simulink model "csthl20_control"  (R2022a)
settings: Solver=ode45  StartTime=0.0  StopTime=80  RelTol=1e-3  EnableMultiTasking=on
PreLoadFcn:
  | % Bus objects
  | load csthl20_BusData
  | 
  | % Controller configuration
  | CTYPE=1;
model workspace (MAT data in the model file):
  A_matrix = [-0.028840208852 -0.0156596305643 -0.0560912779756 -0.0863202941854 0.0209519994416 0.0112571762889 0 0 0 0 0 0 ... (11560 elements, 17x17x8x5)]
  Act2Aero = [0.5 0.5 0 0 0 0 -0.5 0.5 0 0 0 0 ... (42 elements, 6x7)]
  Aero2Act = [1 -1 0 0 0 0 0 1 1 0 0 0 ... (42 elements, 7x6)]
  Aimpoint = 0
  B_matrix = [0 0 0 0 0 0 4 0 0 0 0 0 ... (2040 elements, 17x3x8x5)]
  CX0 = [-0.038092388 -0.040074629 -0.041654124 -0.043173149 -0.044873204 -0.046895013 -0.049278524 -0.051962909 -0.054786564 -0.057487109 -0.059701388 -0.057487109 ... (861 elements, 21x41)]
  CXda = [0.0003742 1.961503e-05 -0.00027008192 -0.00050147477 -0.00068084192 -0.00081415625 -0.00090708512 -0.00096499037 -0.00099292832 -0.00099564977 -0.0009776 -0.00094291877 ... (41 elements, 41x1)]
  CXddf = [0.00027645 0.00032803699 0.00037408304 0.00041515629 0.00045179224 0.00048449375 0.00051373104 0.00053994169 0.00056353064 0.00058487019 0.0006043 0.00062212709 ... (41 elements, 41x1)]
  CXde = [0.00044324 0.000381836538 0.000331656768 0.000291344258 0.000259608768 0.00023522625 0.000217038848 0.000203954898 0.000194948928 0.000189061658 0.0001854 0.000183137058 ... (41 elements, 41x1)]
  CXdfn = [0.00044751 0.0004427177 0.0004388568 0.0004359273 0.0004339292 0.0004328625 0.0004327272 0.0004335233 0.0004352508 0.0004379097 0.0004415 0.0004460217 ... (41 elements, 41x1)]
  CXdfp = [-0.0001151958 -0.000116790098 -0.000118381312 -0.000119969442 -0.000121554488 -0.00012313645 -0.000124715328 -0.000126291122 -0.000127863832 -0.000129433458 -0.000131 -0.000132563458 ... (41 elements, 41x1)]
  CXdr = [0.00020501 3.1047221e-05 -0.000113321344 -0.000231591139 -0.000327061744 -0.000402836875 -0.000461824384 -0.000506736259 -0.000540088624 -0.000564201739 -0.0005812 -0.000593011939 ... (41 elements, 41x1)]
  CYbeta = -0.01242
  CYda = [0.003136571 0.0031983806691 0.0032503278976 0.0032928109331 0.0033262201776 0.0033509381875 0.0033673396736 0.0033757915011 0.0033766526896 0.0033702744131 0.003357 0.0033371649331 ... (41 elements, 41x1)]
  CYddf = [0.000435181 0.0003943016261 0.0003529648896 0.0003113622901 0.0002696754896 0.0002280763125 0.0001867267456 0.0001457789381 0.0001053752016 6.56480101e-05 2.672e-05 -1.12960299e-05 ... (41 elements, 41x1)]
  CYdr = [0.00252708114 0.00237481862595 0.00224430427494 0.00213447047171 0.00204424955574 0.00197257382125 0.00191837551718 0.00188058684723 0.00185813996982 0.00184996699811 0.001855 0.00187217099811 ... (41 elements, 41x1)]
  CZ0 = [0.4485479 0.452540024 0.457747164 0.464172584 0.471737564 0.4802814 0.489561404 0.499252904 0.508949244 0.518161784 0.5263199 0.518161784 ... (861 elements, 21x41)]
  CZda = [0.00078435 0.000747062965 0.00070172464 0.000650226765 0.00059433784 0.000535703125 0.00047584464 0.000416161165 0.00035792824 0.000302298165 0.0002503 0.000202839565 ... (41 elements, 41x1)]
  CZde = [-0.004135092 -0.004296890179 -0.00444395712 -0.004576811367 -0.004695912448 -0.004801660875 -0.004894398144 -0.004974406735 -0.005041910112 -0.005097072723 -0.00514 -0.005170738359 ... (41 elements, 41x1)]
  CZdfn = [-0.00344578 -0.003560437128 -0.003648409408 -0.003712592248 -0.003755747808 -0.003780505 -0.003789359488 -0.003784673688 -0.003768676768 -0.003743464648 -0.003711 -0.003673112248 ... (41 elements, 41x1)]
  CZdfp = [-0.003786031 -0.00378532664 -0.00378462256 -0.00378391876 -0.00378321524 -0.003782512 -0.00378180904 -0.00378110636 -0.00378040396 -0.00377970184 -0.003779 -0.00377829844 ... (41 elements, 41x1)]
  CZdr = [-0.0005037 -0.00036015136 -0.00026716816 -0.00021701736 -0.00020244976 -0.0002167 -0.00025348656 -0.00030701176 -0.00037196176 -0.00044350656 -0.0005173 -0.00058947976 ... (41 elements, 41x1)]
  C_matrix = [0 0 0 0 0 0 0 0 0 -58.994812472 0 0 ... (2040 elements, 3x17x8x5)]
  Clbeta = -0.00787
  Clda = [0.001932032 0.0020326391442 0.0021237120512 0.0022054993322 0.0022782453312 0.002342190125 0.0023975695232 0.0024446150682 0.0024835540352 0.0025146094322 0.002538 0.0025539402122 ... (41 elements, 41x1)]
  Clddf = [0.0007872 0.000807745996 0.000820040096 0.000825228156 0.000824391616 0.0008185475 0.000808648416 0.000795582556 0.000780173696 0.000763181196 0.0007453 0.000727160636 ... (41 elements, 41x1)]
  Cldr = [0.00131521 0.001082613421 0.000885702656 0.000721130461 0.000585704656 0.000476388125 0.000390298816 0.000324709741 0.000277048976 0.000244899661 0.000226 0.000218243261 ... (41 elements, 41x1)]
  Clp = [-0.498 -0.6 -0.398 -0.579 -0.425 -0.499 -0.649 -0.619 -0.81 -0.872 -2.41]
  Clr = [0.496 0.598 0.84 0.806 0.686 0.572 0.603 0.899 0.957 1.357 4.49]
  Cm0 = [0.0380742 0.038701881 0.039695376 0.040900701 0.042196056 0.043491825 0.044730576 0.045887061 0.046968216 0.048013161 0.0490932 0.048013161 ... (861 elements, 21x41)]
  Cmda = [-0.00172492 -0.001358222162 -0.001043014432 -0.000774578842 -0.000548407232 -0.00036020125 -0.000205872352 -8.1541802e-05 1.6459328e-05 9.1590158e-05 0.0001471 0.000186028358 ... (41 elements, 41x1)]
  Cmde = [-0.00155002 -0.001596102826 -0.001641310016 -0.001685002906 -0.001726581856 -0.00176548625 -0.001801194496 -0.001833224026 -0.001861131296 -0.001884511786 -0.001903 -0.001916269466 ... (41 elements, 41x1)]
  Cmdfn = [-0.00114421 -0.001160648097 -0.001169150592 -0.001170952777 -0.001167224592 -0.001159070625 -0.001147530112 -0.001133576937 -0.001118119632 -0.001102001377 -0.001086 -0.001070827977 ... (41 elements, 41x1)]
  Cmdfp = [-0.000989578757 -0.00098958144857 -0.00098958401408 -0.00098958645353 -0.00098958876692 -0.00098959095425 -0.00098959301552 -0.00098959495073 -0.00098959675988 -0.00098959844297 -0.0009896 -0.00098960143097 ... (41 elements, 41x1)]
  Cmdr = [0.000290283 0.0002382539513 0.0001902563968 0.0001463019633 0.0001063833968 7.04745625e-05 3.85304448e-05 1.04871473e-05 -1.37381072e-05 -3.42469767e-05 -5.116e-05 -6.46165967e-05 ... (41 elements, 41x1)]
  Cmq = [-0.203 -0.158 -0.116 -0.176 -0.176 -0.175 -0.174 -0.252 -0.299 -0.571 -0.8]
  Cn0 = [0 0 0 0 0 0 0 0 0 0.0046 0.0056 0.01 ... (36 elements, 9x4)]
  Cnda = [-0.00092498 -0.001272671988 -0.001576223168 -0.001838775908 -0.002063359968 -0.0022528925 -0.002410178048 -0.002537908548 -0.002638663328 -0.002714909108 -0.002769 -0.002803177508 ... (41 elements, 41x1)]
  Cnddf = [-0.000146484 -0.0001398019207 -0.0001321750752 -0.0001237254087 -0.0001145714752 -0.0001048284375 -9.46080672e-05 -8.40187447e-05 -7.31654592e-05 -6.21498087e-05 -5.107e-05 -4.00208487e-05 ... (41 elements, 41x1)]
  Cndr = [-0.0021525 -0.00197387964 -0.00182075584 -0.00169102464 -0.00158266224 -0.001493725 -0.00142234944 -0.00136675224 -0.00132523024 -0.00129616044 -0.001278 -0.00126928624 ... (41 elements, 41x1)]
  Cnp = [0.381 0.353 0.219 0.244 0.179 0.167 0.201 0.222 0.307 0.379 0.85]
  Cnr = [-0.794 -0.837 -0.921 -0.922 -0.867 -0.922 -0.946 -1.007 -1.09 -1.286 -2.041]
  Euler_0 = [0; -0.199448681609; 0.174532925199]
  F_matrix = [5.97622599319 0.726116013193 -2.64604157338 40.7494939461 -11.661494324 -21.0342779763 -20.6745716213 19.9416021106 13.12545371 -926.002157715 187.969629212 231.434488107 ... (2040 elements, 3x17x8x5)]
  H_matrix = [-0.0157218860845 -0.283968320777 0.321370128412 0.271058535159 0.0185568065093 -0.00784369239396 -0.320886300542 1.82463546416 -0.0471251877299 0.142152392032 -0.0609086167769 0.505612659091 ... (2040 elements, 17x3x8x5)]
  Inertia = [12429.9503379  0  0; 0  72478.3946274  0; 0  0  72478.3946274]
  Ixx = 12429.9503379
  Iyy = 72478.3946274
  Izz = 72478.3946274
  Kalpha = [0.0423424456751 0.0568591289308 0.102067434202 0.0770570952411 0.0850957010804 0.0662889030912 0.0515945392978 0.0567349800611 0.0609882520612 0.0639334226074 0.102956303686 0.0735712249771 ... (40 elements, 8x5)]
  Kalpha_1 = [0.0675525766417; 0.0670941520285; 0.105277724217; 0.0705938909254; 0.0692391670282; 0.0682506457138; 0.0672739862702; 0.0668102273189]
  Kbeta = [-0.0421966217034 -0.0316770241418 -0.0293493744968 -0.0256527675357 -0.0307095576987 -0.0325234533837 -0.0335699630482 -0.0320760010348 -0.034523712176 -0.0332114192463 -0.0353203051713 -0.0341700804254 ... (40 elements, 8x5)]
  Kbeta_1 = [-0.0493656538568; -0.0419788515038; -0.0374619432887; -0.0381850673629; -0.0395050518916; -0.0416555062349; -0.0442775778109; -0.0483706672557]
  Kg2lb = 2.20462
  Kg2slug = 0.0685218
  Ki33 = [0.05 0 0 0 0.05 0 0 0 -0.05 0.05 0 0 ... (360 elements, 3x3x8x5)]
  Kp = [58.994812472 52.4118047689 51.4724972494 52.6814724048 55.5352541837 58.9018334743 63.6260316602 72.5872875233 59.9420490209 52.6642968779 51.592012551 53.0773749012 ... (40 elements, 8x5)]
  Kp_1 = [60.2253428509; 52.7939261692; 51.6224369342; 53.1835874806; 55.9559014793; 59.5393657693; 64.8225348547; 75.6927037235]
  Kphi = [0.0897851430865 0.0905292361524 0.0908849236023 0.0911263381707 0.0895187966623 0.0900454862025 0.0906744952369 0.0929073813074 0.0903130708487 0.090501875878 0.0906948768638 0.0909697583395 ... (40 elements, 8x5)]
  Kphi_1 = [0.0899736559878; 0.0903144259517; 0.0907381573489; 0.0909707194509; 0.0897040590713; 0.0897346237436; 0.0909239286068; 0.092390635977]
  Kq = [-180.388522844 -183.274455652 -174.601566615 -173.806564517 -181.332040221 -198.869769941 -229.860472425 -279.151066798 -195.144174655 -181.815188811 -174.318203455 -173.650391198 ... (40 elements, 8x5)]
  Kq_1 = [-190.665384898; -180.322553126; -174.03272401; -173.493656781; -180.877109643; -197.917252796; -228.270830002; -278.51108854]
  Kr = [-713.893478208 -1002.12341186 -1153.7416491 -1153.7295441 -1077.83714501 -1007.5234901 -1017.22971433 -1059.1938939 -717.84572737 -1002.7104968 -1155.32550182 -1152.14420545 ... (40 elements, 8x5)]
  Kr_1 = [-714.366713062; -1002.72404317; -1151.4783324; -1152.96908365; -1070.59786805; -1009.08046077; -1000.48966647; -1058.93322007]
  L = 0.0065
  P0 = 101325
  PolyCoeff = [0.0005173 7.359e-05 -8.27e-07 -6.034e-07 2.016e-08 -5.116e-05 -1.516e-05 1.729e-06 -2.481e-08 -7.867e-10 0.0005812 1.41e-05 ... (30 elements, 5x6)]
  R = 287.26
  S_ref = 26.6120741048
  T0 = 288.16
  Tc : Simulink.Parameter (value not decoded)
  Tf = 0.0333333333333
  U_trim_matrix = [-23.7683817467 -4.33440943636 4.43733647183 -22.1955716586 4.52075664841 21.6532360323 -20.4783849922 6.34956743865 19.7065472455 -22.2662158495 5.88613316784 30.8883374276 ... (120 elements, 3x8x5)]
  V = 204
  Vmw = [202.669961421; 0; 23.256971809]
  Xglide = [0 50 100 150 200 250 300 350 400 450 500 550 ... (301 elements, 1x301)]
  a_matrix = [-0.028840208852 -0.0156596305643 -0.0560912779756 -0.0863202941854 0.0209519994416 0.0112571762889 23.9049039727 0 2.90446405277 0 -10.5841662935 0 ... (11560 elements, 17x17x8x5)]
  a_matrix_r = [-156.820455268 -2.6081545927 7.98280879857 -52.6889464944 -98.7536402844 -31.0538337205 -56.8560446475 -13.5355572892 20.9647022526 5.44178466439 10.8726065796 -74.0228373916 ... (4000 elements, 10x10x8x5)]
  a_vec = [-10 -5 0 5 10 15 20 25]
  al = [-10 -10 -10 -10 -10 -10 -10 -10 -10 -10 -10 -10 ... (861 elements, 861x1)]
  alpha0 = 0.114253174362
  alpha_0 = 0.114253174362
  alpha_vec_0 = [-10 -9 -8 -7 -6 -5 -4 -3 -2 -1 0 1 ... (41 elements, 1x41)]
  alpha_vec_Cn0 = [-10 -5 0 5 10 15 20 25 30]
  alpha_vec_damping = [0 5 10 12 14 16 18 20 22 25 30]
  b_matrix = [-0.0157218860845 -0.283968320777 0.321370128412 0.271058535159 0.0185568065093 -0.00784369239396 -0.320886300542 1.82463546416 -0.0471251877299 0.142152392032 -0.0609086167769 0.505612659091 ... (2040 elements, 17x3x8x5)]
  b_matrix_r = [16.1920898553 5.30458121646 -0.595159501787 0.926408673902 1.71445620697 0.355342126068 0.32457458722 0.685332204474 -1.16437558272 -0.29270115931 -11.0077968955 7.7054244731 ... (1200 elements, 10x3x8x5)]
  b_ref = 4.23367186452
  b_vec = [-10 -5 0 5 10]
  be = [-10 -9 -8 -7 -6 -5 -4 -3 -2 -1 0 1 ... (861 elements, 861x1)]
  beta_vec_0 = [-10 -9 -8 -7 -6 -5 -4 -3 -2 -1 0 1 ... (21 elements, 1x21)]
  beta_vec_Cn0 = [0 2 5 10]
  c_matrix = [-5.97622599319 -0.726116013193 2.64604157338 -40.7494939461 11.661494324 21.0342779763 20.6745716213 -19.9416021106 -13.12545371 926.002157715 -187.969629212 -231.434488107 ... (2040 elements, 3x17x8x5)]
  c_matrix_r = [15.2602338676 -5.43568873341 -5.10812577276 3.18529730179 7.88989001471 2.44811627957 -2.14984449181 2.50002941397 -6.57393218937 -0.387383577292 0.599324432144 0.592603066114 ... (1200 elements, 3x10x8x5)]
  d2r = 0.0174532925199
  d_matrix = [0 0 0 0 0 0 0 0 0 0 0 0 ... (360 elements, 3x3x8x5)]
  d_matrix_r = [0.0645179305383 -0.0277031296271 0.00912008654979 -0.026123256393 0.0358025045637 -0.00303736235544 0.00773298157175 0.0154534545894 0.0234258693594 0.0641966240952 -0.0199541298617 1.95187006231e-05 ... (360 elements, 3x3x8x5)]
  d_ref = 8.60755172456
  dbf_max = 60
  den_g = [1 -0.860465116279]
  dr_max = 60
  dwf_max = 30
  g = 9.81
  gam = 1.403
  gamma1 = 0.313701855971
  h_trop = 11000
  hglide = [0 2.62038896415 5.2407779283 7.86116689246 10.4815558566 13.1019448208 15.7223337849 18.3427227491 20.9631117132 23.5835006774 26.2038896415 28.8242786057 ... (301 elements, 1x301)]
  len_veh = 8.32408773363
  m2ft = 3.28084
  mass = 11738.9844962
  massBody = 10401.7925992
  massFuel = 1337.19189702
  max_lim = [30 30 60 60 0 0 60]
  min_lim = [-30 -30 0 0 -60 -60 -60]
  num_g = [0.930930232558 -0.929534883721]
  pm_0 = [0; 0; 0]
  qbar0 = 10722.8924586
  rho0 = 1.225
  temp = [0.0005037 0.00036015136 0.00026716816 0.00021701736 0.00020244976 0.0002167 0.00025348656 0.00030701176 0.00037196176 0.00044350656 0.0005173 0.00058947976 ... (246 elements, 41x6)]
  ts = 0.01
  wn_act = 44
  x_cg = 4.78635044684
  x_ref = 4.49500737616
  xme_0 = [-12071.9115088; -1000; -3047.99990246]
  z_act = 0.707106781187
symbols that are objects in the model workspace (value not decoded): Tc
undefined symbols (not defined in the file or in its folder): DiscIntNeverNeededParam, ft, m, s
libraries: discretizing x10, aerolibconvert2 x4, slpidlib x3, aerolibconvert x2, simulink_extras x1, csthl20_lib x1, simulink x1
(part 3 of 3)

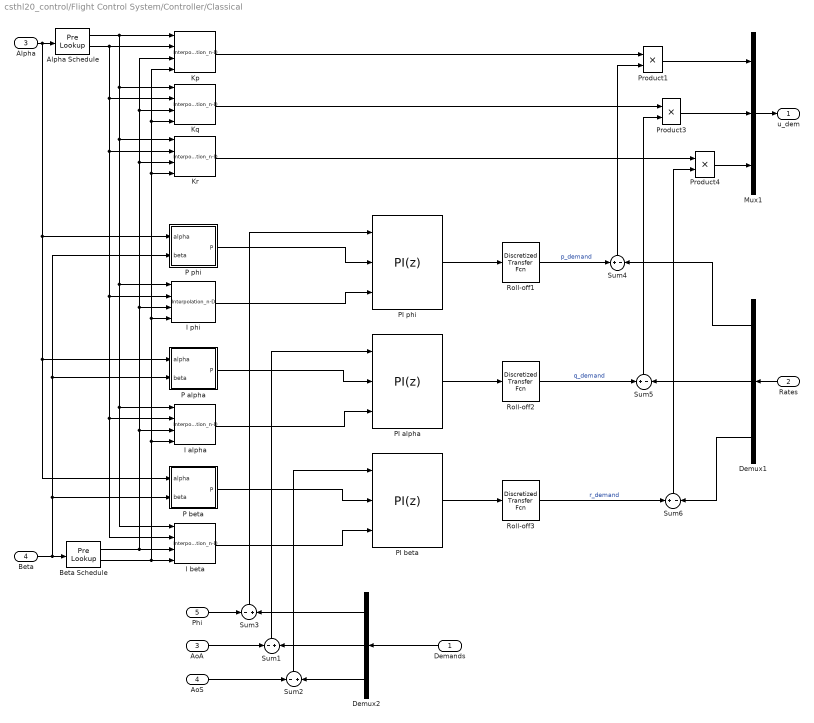
== system csthl20_control/Flight Control System/Controller/Classical ==
  Demands : Inport  PortDimensions=3
  Rates : Inport  Port=2  PortDimensions=3
  AoA : Inport  Port=3  PortDimensions=1
  AoS : Inport  Port=4  PortDimensions=1
  Phi : Inport  Port=5  PortDimensions=1
  Alpha : InportShadow  Port=3  PortDimensions=1
  Alpha Schedule : PreLookup  BreakpointsData=a_vec  BeginIndexSearchUsingPreviousIndexResult=on  ExtrapMethod=Linear
  Beta : InportShadow  Port=4  PortDimensions=1
  Beta Schedule : PreLookup  BreakpointsData=b_vec  BeginIndexSearchUsingPreviousIndexResult=on  ExtrapMethod=Linear
  Demux1 : Demux  Outputs=3
      settings: DisplayOption=none
  Demux2 : Demux  Outputs=3
      settings: DisplayOption=none
  I alpha : Interpolation_n-D  Table=Kalpha  RemoveProtectionIndex=on
  I beta : Interpolation_n-D  Table=Kbeta  RemoveProtectionIndex=on
  I phi : Interpolation_n-D  Table=Kphi  RemoveProtectionIndex=on
  Kp : Interpolation_n-D  Table=Kp  RemoveProtectionIndex=on
  Kq : Interpolation_n-D  Table=Kq  RemoveProtectionIndex=on
  Kr : Interpolation_n-D  Table=Kr  RemoveProtectionIndex=on
  Mux1 : Mux  Inputs=3
  P alpha : MATLAB Function  TreatAsAtomicUnit=on
  P beta : MATLAB Function  TreatAsAtomicUnit=on
  P phi : MATLAB Function  TreatAsAtomicUnit=on
  PI alpha : slpidlib/PID Controller  Controller=PI  Form=Parallel  TimeDomain=Discrete-time  UseExternalTs=off  SampleTime=Tc  IntegratorMethod=Forward Euler  FilterMethod=Forward Euler  ControllerParametersSource=external  P=1  I=1  UseKiTs=off  D=0  N=100  UseFilter=on  TunerSelectOption=Transfer Function Based (PID Tuner App)  InitialConditionSource=internal  InitialConditionForIntegrator=0  InitialConditionForFilter=0  DifferentiatorICPrevScaledInput=0  ExternalReset=none  TrackingMode=off  Kt=1  LimitOutput=off  SatLimitsSource=internal  UpperSaturationLimit=inf  LowerSaturationLimit=-inf  LinearizeAsGain=off  AntiWindupMode=none  Kb=1  POutMin=[]  POutMax=[]  IOutMin=[]  IOutMax=[]  DOutMin=[]  DOutMax=[]  NOutMin=[]  NOutMax=[]  SumOutMin=[]  SumOutMax=[]  SaturationOutMin=[]  SaturationOutMax=[]  PParamMin=[]  PParamMax=[]  IParamMin=[]  IParamMax=[]  DParamMin=[]  DParamMax=[]  NParamMin=[]  NParamMax=[]  KbParamMin=[]  KbParamMax=[]  KtParamMin=[]  KtParamMax=[]  KbOutMin=[]  KbOutMax=[]  KtOutMin=[]  KtOutMax=[]  IntegratorOutMin=[]  IntegratorOutMax=[]  FilterOutMin=[]  FilterOutMax=[]  SumI1OutMin=[]  SumI1OutMax=[]  SumI2OutMin=[]  SumI2OutMax=[]  SumI3OutMin=[]  SumI3OutMax=[]  SumI4OutMin=[]  SumI4OutMax=[]  SumDOutMin=[]  SumDOutMax=[]  DifferentiatorOutMin=[]  DifferentiatorOutMax=[]  FilterDiffOutCoefMin=[]  FilterDiffOutCoefMax=[]  ReciprocalOutMin=[]  ReciprocalOutMax=[]  SumDenOutMin=[]  SumDenOutMax=[]  SumNumOutMin=[]  SumNumOutMax=[]  DivideOutMin=[]  DivideOutMax=[]  UdiffTsProdOutMin=[]  UdiffTsProdOutMax=[]  NTsProdOutMin=[]  NTsProdOutMax=[]  UintegralTsProdOutMin=[]  UintegralTsProdOutMax=[]  UngainTsProdOutMin=[]  UngainTsProdOutMax=[]  IntegratorContinuousStateAttributes=''  IntegratorStateMustResolveToSignalObject=off  IntegratorRTWStateStorageClass=Auto  FilterContinuousStateAttributes=''  FilterStateMustResolveToSignalObject=off  FilterRTWStateStorageClass=Auto  ParallelPVariant=ExternalParameters  IdealPVariant=Disabled  IVariant=ExternalParameters  DVariant=Disabled  IntegratorVariant=Discrete  SatVariant=Disabled  AWVariant=Passthrough  PCopyVariant=Disabled  TRVariant=Disabled  FdbkBlocksVariant=Forward  IdealPFdbkVariant=Disabled  SatFdbkVariant=Disabled  DerivativeFilterVariant=Disabled  NVariant=Disabled  NCopyVariant=Disabled_SignalSpec  FilterICVariant=Disabled  IntegratorICVariant=InternalICs  ExternalResetVariant=Disabled  TRSumVariant=Passthrough  SumFdbkVariant=Disabled  SumVariant=Sum_PI  TsampFilterVariant=InternalTs  TsampNgainVariant=Passthrough  TsampIntegralVariant=Passthrough  ExternalSaturationOutDataTypeStr=Inherit: Same as second input  aMode=0
  PI beta : slpidlib/PID Controller  Controller=PI  Form=Parallel  TimeDomain=Discrete-time  UseExternalTs=off  SampleTime=Tc  IntegratorMethod=Forward Euler  FilterMethod=Forward Euler  ControllerParametersSource=external  P=1  I=1  UseKiTs=off  D=0  N=100  UseFilter=on  TunerSelectOption=Transfer Function Based (PID Tuner App)  InitialConditionSource=internal  InitialConditionForIntegrator=0  InitialConditionForFilter=0  DifferentiatorICPrevScaledInput=0  ExternalReset=none  TrackingMode=off  Kt=1  LimitOutput=off  SatLimitsSource=internal  UpperSaturationLimit=inf  LowerSaturationLimit=-inf  LinearizeAsGain=off  AntiWindupMode=none  Kb=1  POutMin=[]  POutMax=[]  IOutMin=[]  IOutMax=[]  DOutMin=[]  DOutMax=[]  NOutMin=[]  NOutMax=[]  SumOutMin=[]  SumOutMax=[]  SaturationOutMin=[]  SaturationOutMax=[]  PParamMin=[]  PParamMax=[]  IParamMin=[]  IParamMax=[]  DParamMin=[]  DParamMax=[]  NParamMin=[]  NParamMax=[]  KbParamMin=[]  KbParamMax=[]  KtParamMin=[]  KtParamMax=[]  KbOutMin=[]  KbOutMax=[]  KtOutMin=[]  KtOutMax=[]  IntegratorOutMin=[]  IntegratorOutMax=[]  FilterOutMin=[]  FilterOutMax=[]  SumI1OutMin=[]  SumI1OutMax=[]  SumI2OutMin=[]  SumI2OutMax=[]  SumI3OutMin=[]  SumI3OutMax=[]  SumI4OutMin=[]  SumI4OutMax=[]  SumDOutMin=[]  SumDOutMax=[]  DifferentiatorOutMin=[]  DifferentiatorOutMax=[]  FilterDiffOutCoefMin=[]  FilterDiffOutCoefMax=[]  ReciprocalOutMin=[]  ReciprocalOutMax=[]  SumDenOutMin=[]  SumDenOutMax=[]  SumNumOutMin=[]  SumNumOutMax=[]  DivideOutMin=[]  DivideOutMax=[]  UdiffTsProdOutMin=[]  UdiffTsProdOutMax=[]  NTsProdOutMin=[]  NTsProdOutMax=[]  UintegralTsProdOutMin=[]  UintegralTsProdOutMax=[]  UngainTsProdOutMin=[]  UngainTsProdOutMax=[]  IntegratorContinuousStateAttributes=''  IntegratorStateMustResolveToSignalObject=off  IntegratorRTWStateStorageClass=Auto  FilterContinuousStateAttributes=''  FilterStateMustResolveToSignalObject=off  FilterRTWStateStorageClass=Auto  ParallelPVariant=ExternalParameters  IdealPVariant=Disabled  IVariant=ExternalParameters  DVariant=Disabled  IntegratorVariant=Discrete  SatVariant=Disabled  AWVariant=Passthrough  PCopyVariant=Disabled  TRVariant=Disabled  FdbkBlocksVariant=Forward  IdealPFdbkVariant=Disabled  SatFdbkVariant=Disabled  DerivativeFilterVariant=Disabled  NVariant=Disabled  NCopyVariant=Disabled_SignalSpec  FilterICVariant=Disabled  IntegratorICVariant=InternalICs  ExternalResetVariant=Disabled  TRSumVariant=Passthrough  SumFdbkVariant=Disabled  SumVariant=Sum_PI  TsampFilterVariant=InternalTs  TsampNgainVariant=Passthrough  TsampIntegralVariant=Passthrough  ExternalSaturationOutDataTypeStr=Inherit: Same as second input  aMode=0
  PI phi : slpidlib/PID Controller  Controller=PI  Form=Parallel  TimeDomain=Discrete-time  UseExternalTs=off  SampleTime=Tc  IntegratorMethod=Forward Euler  FilterMethod=Forward Euler  ControllerParametersSource=external  P=1  I=1  UseKiTs=off  D=0  N=100  UseFilter=on  TunerSelectOption=Transfer Function Based (PID Tuner App)  InitialConditionSource=internal  InitialConditionForIntegrator=0  InitialConditionForFilter=0  DifferentiatorICPrevScaledInput=0  ExternalReset=none  TrackingMode=off  Kt=1  LimitOutput=off  SatLimitsSource=internal  UpperSaturationLimit=inf  LowerSaturationLimit=-inf  LinearizeAsGain=off  AntiWindupMode=none  Kb=1  POutMin=[]  POutMax=[]  IOutMin=[]  IOutMax=[]  DOutMin=[]  DOutMax=[]  NOutMin=[]  NOutMax=[]  SumOutMin=[]  SumOutMax=[]  SaturationOutMin=[]  SaturationOutMax=[]  PParamMin=[]  PParamMax=[]  IParamMin=[]  IParamMax=[]  DParamMin=[]  DParamMax=[]  NParamMin=[]  NParamMax=[]  KbParamMin=[]  KbParamMax=[]  KtParamMin=[]  KtParamMax=[]  KbOutMin=[]  KbOutMax=[]  KtOutMin=[]  KtOutMax=[]  IntegratorOutMin=[]  IntegratorOutMax=[]  FilterOutMin=[]  FilterOutMax=[]  SumI1OutMin=[]  SumI1OutMax=[]  SumI2OutMin=[]  SumI2OutMax=[]  SumI3OutMin=[]  SumI3OutMax=[]  SumI4OutMin=[]  SumI4OutMax=[]  SumDOutMin=[]  SumDOutMax=[]  DifferentiatorOutMin=[]  DifferentiatorOutMax=[]  FilterDiffOutCoefMin=[]  FilterDiffOutCoefMax=[]  ReciprocalOutMin=[]  ReciprocalOutMax=[]  SumDenOutMin=[]  SumDenOutMax=[]  SumNumOutMin=[]  SumNumOutMax=[]  DivideOutMin=[]  DivideOutMax=[]  UdiffTsProdOutMin=[]  UdiffTsProdOutMax=[]  NTsProdOutMin=[]  NTsProdOutMax=[]  UintegralTsProdOutMin=[]  UintegralTsProdOutMax=[]  UngainTsProdOutMin=[]  UngainTsProdOutMax=[]  IntegratorContinuousStateAttributes=''  IntegratorStateMustResolveToSignalObject=off  IntegratorRTWStateStorageClass=Auto  FilterContinuousStateAttributes=''  FilterStateMustResolveToSignalObject=off  FilterRTWStateStorageClass=Auto  ParallelPVariant=ExternalParameters  IdealPVariant=Disabled  IVariant=ExternalParameters  DVariant=Disabled  IntegratorVariant=Discrete  SatVariant=Disabled  AWVariant=Passthrough  PCopyVariant=Disabled  TRVariant=Disabled  FdbkBlocksVariant=Forward  IdealPFdbkVariant=Disabled  SatFdbkVariant=Disabled  DerivativeFilterVariant=Disabled  NVariant=Disabled  NCopyVariant=Disabled_SignalSpec  FilterICVariant=Disabled  IntegratorICVariant=InternalICs  ExternalResetVariant=Disabled  TRSumVariant=Passthrough  SumFdbkVariant=Disabled  SumVariant=Sum_PI  TsampFilterVariant=InternalTs  TsampNgainVariant=Passthrough  TsampIntegralVariant=Passthrough  ExternalSaturationOutDataTypeStr=Inherit: Same as second input  aMode=0
  Product1 : Product  InputSameDT=on  SaturateOnIntegerOverflow=on  OutDataTypeStr=Inherit: Same as first input
  Product3 : Product  InputSameDT=on  SaturateOnIntegerOverflow=on  OutDataTypeStr=Inherit: Same as first input
  Product4 : Product  InputSameDT=on  SaturateOnIntegerOverflow=on  OutDataTypeStr=Inherit: Same as first input
  Roll-off1 : discretizing/Discretized Transfer Fcn  Numerator=10  Denominator=[1, 10]  AbsTol=auto  SampleTime=Tc  method=zoh  Wc=1
      settings: SourceProductBaseCode=SL
  Roll-off2 : discretizing/Discretized Transfer Fcn  Numerator=10  Denominator=[1, 10]  AbsTol=auto  SampleTime=Tc  method=zoh  Wc=1
      settings: SourceProductBaseCode=SL
  Roll-off3 : discretizing/Discretized Transfer Fcn  Numerator=10  Denominator=[1, 10]  AbsTol=auto  SampleTime=Tc  method=zoh  Wc=1
      settings: SourceProductBaseCode=SL
  Sum1 : Sum  Inputs=-|+  InputSameDT=on  SaturateOnIntegerOverflow=on  OutDataTypeStr=Inherit: Same as first input
  Sum2 : Sum  Inputs=-|+  InputSameDT=on  SaturateOnIntegerOverflow=on  OutDataTypeStr=Inherit: Same as first input
  Sum3 : Sum  Inputs=-|+  InputSameDT=on  SaturateOnIntegerOverflow=on  OutDataTypeStr=Inherit: Same as first input
  Sum4 : Sum  Inputs=+|-  InputSameDT=on  SaturateOnIntegerOverflow=on  OutDataTypeStr=Inherit: Same as first input
  Sum5 : Sum  Inputs=+|-  InputSameDT=on  SaturateOnIntegerOverflow=on  OutDataTypeStr=Inherit: Same as first input
  Sum6 : Sum  Inputs=+|-  InputSameDT=on  SaturateOnIntegerOverflow=on  OutDataTypeStr=Inherit: Same as first input
  u_dem : Outport  InitialOutput=[0 0 0]  VectorParamsAs1DForOutWhenUnconnected=off
  wires:
  Beta Schedule/2 -> I beta/4, Kp/4, Kq/4, Kr/4, I phi/4, I alpha/4
  Beta Schedule/1 -> Kr/3, Kp/3, Kq/3, I phi/3, I alpha/3, I beta/3
  Beta/1 -> Beta Schedule/1, P beta/2(beta), P alpha/2(beta), P phi/2(beta)
  Alpha Schedule/2 -> Kp/2, Kq/2, I beta/2, I alpha/2, I phi/2, Kr/2
  Alpha Schedule/1 -> Kp/1, I beta/1, I alpha/1, I phi/1, Kr/1, Kq/1
  Alpha/1 -> P beta/1(alpha), P alpha/1(alpha), P phi/1(alpha), Alpha Schedule/1
  Roll-off1/1 -> Sum4/1  "p_demand"
  PI beta/1 -> Roll-off3/1
  Roll-off2/1 -> Sum5/1  "q_demand"
  Roll-off3/1 -> Sum6/1  "r_demand"
  Demux2/1 -> Sum3/2
  Sum4/1 -> Product1/2
  Kr/1 -> Product4/1
  Kp/1 -> Product1/1
  Kq/1 -> Product3/1
  Rates/1 -> Demux1/1
  Demux1/1 -> Sum4/2
  Demux1/2 -> Sum5/2
  Demux1/3 -> Sum6/2
  Mux1/1 -> u_dem/1
  Product1/1 -> Mux1/1
  Product3/1 -> Mux1/2
  Sum5/1 -> Product3/2
  Product4/1 -> Mux1/3
  Sum6/1 -> Product4/2
  PI phi/1 -> Roll-off1/1
  P phi/1(P) -> PI phi/2
  I phi/1 -> PI phi/3
  P alpha/1(P) -> PI alpha/2
  I alpha/1 -> PI alpha/3
  PI alpha/1 -> Roll-off2/1
  P beta/1(P) -> PI beta/2
  I beta/1 -> PI beta/3
  Demux2/2 -> Sum1/2
  Phi/1 -> Sum3/1
  Sum3/1 -> PI phi/1
  Sum1/1 -> PI alpha/1
  AoA/1 -> Sum1/1
  Demux2/3 -> Sum2/2
  AoS/1 -> Sum2/1
  Sum2/1 -> PI beta/1
  Demands/1 -> Demux2/1

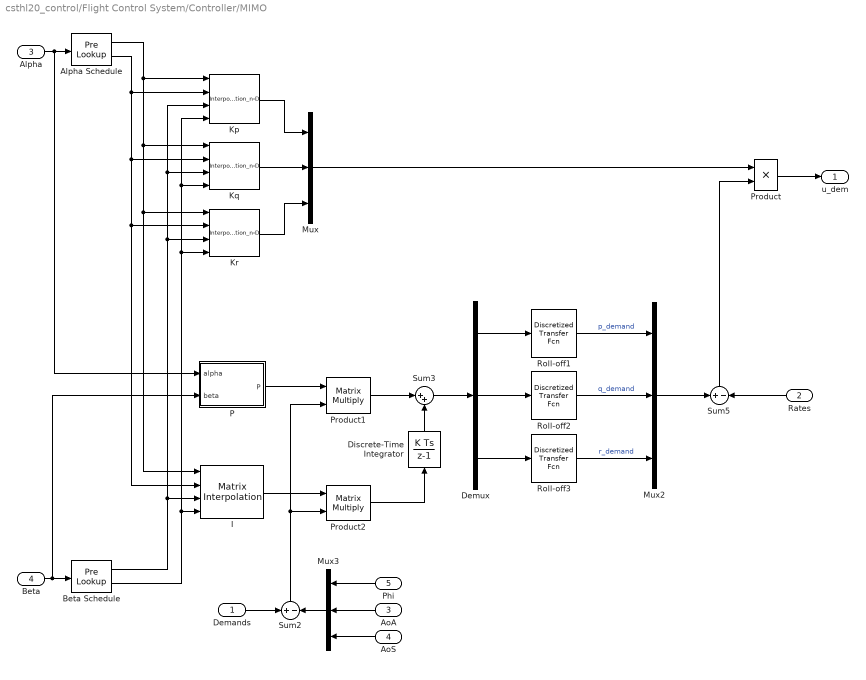
== system csthl20_control/Flight Control System/Controller/MIMO ==
  Demands : Inport  PortDimensions=3
  Rates : Inport  Port=2  PortDimensions=3
  AoA : Inport  Port=3  PortDimensions=1
  AoS : Inport  Port=4  PortDimensions=1
  Phi : Inport  Port=5  PortDimensions=1
  Alpha : InportShadow  Port=3  PortDimensions=1
  Alpha Schedule : PreLookup  BreakpointsData=a_vec  BeginIndexSearchUsingPreviousIndexResult=on  ExtrapMethod=Linear
  Beta : InportShadow  Port=4  PortDimensions=1
  Beta Schedule : PreLookup  BreakpointsData=b_vec  BeginIndexSearchUsingPreviousIndexResult=on  ExtrapMethod=Linear
  Demux : Demux  Outputs=3
      settings: DisplayOption=none
  Discrete-Time Integrator : DiscreteIntegrator  SampleTime=Tc  ICPrevOutput=DiscIntNeverNeededParam  ICPrevScaledInput=DiscIntNeverNeededParam
  I : simulink_extras/Additional Lookup Tables/Matrix Interpolation  InterpMethod=Linear  ExtrapMethod=Clip  InterpolateDimension=2  TableData=Ki33  SimulateUsing=Interpreted execution
      settings: SourceProductBaseCode=SL
  Kp : Interpolation_n-D  Table=Kp  RemoveProtectionIndex=on
  Kq : Interpolation_n-D  Table=Kq  RemoveProtectionIndex=on
  Kr : Interpolation_n-D  Table=Kr  RemoveProtectionIndex=on
  Mux : Mux  Inputs=[1,1,1]
  Mux2 : Mux  Inputs=[1,1,1]
  Mux3 : Mux  Inputs=[1,1,1]
  P : MATLAB Function  TreatAsAtomicUnit=on
  Product : Product  InputSameDT=on  SaturateOnIntegerOverflow=on  OutDataTypeStr=Inherit: Same as first input
  Product1 : Product  Multiplication=Matrix(*)  InputSameDT=on  SaturateOnIntegerOverflow=on  OutDataTypeStr=Inherit: Same as first input
  Product2 : Product  Multiplication=Matrix(*)  InputSameDT=on  SaturateOnIntegerOverflow=on  OutDataTypeStr=Inherit: Same as first input
  Roll-off1 : discretizing/Discretized Transfer Fcn  Numerator=10  Denominator=[1, 10]  AbsTol=auto  SampleTime=Tc  method=zoh  Wc=1
      settings: SourceProductBaseCode=SL
  Roll-off2 : discretizing/Discretized Transfer Fcn  Numerator=10  Denominator=[1, 10]  AbsTol=auto  SampleTime=Tc  method=zoh  Wc=1
      settings: SourceProductBaseCode=SL
  Roll-off3 : discretizing/Discretized Transfer Fcn  Numerator=10  Denominator=[1, 10]  AbsTol=auto  SampleTime=Tc  method=zoh  Wc=1
      settings: SourceProductBaseCode=SL
  Sum2 : Sum  Inputs=+|-  InputSameDT=on  SaturateOnIntegerOverflow=on  OutDataTypeStr=Inherit: Same as first input
  Sum3 : Sum  Inputs=|++  InputSameDT=on  SaturateOnIntegerOverflow=on  OutDataTypeStr=Inherit: Same as first input
  Sum5 : Sum  Inputs=+|-  InputSameDT=on  SaturateOnIntegerOverflow=on  OutDataTypeStr=Inherit: Same as first input
  u_dem : Outport  InitialOutput=[0 0 0]  VectorParamsAs1DForOutWhenUnconnected=off
  wires:
  Sum3/1 -> Demux/1
  Demux/2 -> Roll-off2/1
  Demux/1 -> Roll-off1/1
  Sum2/1 -> Product1/2, Product2/2
  I/1 -> Product2/1
  Phi/1 -> Mux3/1
  AoA/1 -> Mux3/2
  AoS/1 -> Mux3/3
  Mux3/1 -> Sum2/2
  Beta Schedule/2 -> I/4, Kq/4, Kp/4, Kr/4
  Beta Schedule/1 -> I/3, Kr/3, Kp/3, Kq/3
  Beta/1 -> P/2(beta), Beta Schedule/1
  Alpha Schedule/2 -> Kp/2, Kq/2, I/2, Kr/2
  Alpha Schedule/1 -> I/1, Kr/1, Kq/1, Kp/1
  Alpha/1 -> Alpha Schedule/1, P/1(alpha)
  Product2/1 -> Discrete-Time Integrator/1
  Discrete-Time Integrator/1 -> Sum3/2
  Product1/1 -> Sum3/1
  Roll-off1/1 -> Mux2/1  "p_demand"
  Demux/3 -> Roll-off3/1
  Roll-off2/1 -> Mux2/2  "q_demand"
  Roll-off3/1 -> Mux2/3  "r_demand"
  Demands/1 -> Sum2/1
  P/1(P) -> Product1/1
  Rates/1 -> Sum5/2
  Sum5/1 -> Product/2
  Mux/1 -> Product/1
  Product/1 -> u_dem/1
  Kp/1 -> Mux/1
  Kq/1 -> Mux/2
  Kr/1 -> Mux/3
  Mux2/1 -> Sum5/1

== system csthl20_control/Guidance System/Guide to Glideslope/Low Pass ==
  In1 : Inport
  Discrete-Time Integrator : DiscreteIntegrator  InitialConditionSource=external  SampleTime=ts  ICPrevOutput=DiscIntNeverNeededParam  ICPrevScaledInput=DiscIntNeverNeededParam
  Omega : Gain  Gain=2  SaturateOnIntegerOverflow=on  OutDataTypeStr=Inherit: Same as input  ParamDataTypeStr=Inherit: Same as input
  Sum3 : Sum  Inputs=|+-  InputSameDT=on  SaturateOnIntegerOverflow=on  OutDataTypeStr=Inherit: Same as first input
  Out1 : Outport  VectorParamsAs1DForOutWhenUnconnected=off
  wires:
  In1/1 -> Discrete-Time Integrator/2, Sum3/1
  Discrete-Time Integrator/1 -> Out1/1, Sum3/2
  Sum3/1 -> Omega/1
  Omega/1 -> Discrete-Time Integrator/1

== matlab function csthl20_control/Flight Control System/Controller/Classical/P phi ==
  data: alpha input; P output; beta input
function P = fcn(alpha,beta)

P = 0.05;

== matlab function csthl20_control/Flight Control System/Controller/Classical/P alpha ==
  data: alpha input; P output; beta input
function P = fcn(alpha,beta)

P = 0.05;

== matlab function csthl20_control/Flight Control System/Controller/Classical/P beta ==
  data: alpha input; P output; beta input
function P = fcn(alpha,beta)

P = -0.05;

== matlab function csthl20_control/Flight Control System/Controller/MIMO/P ==
  data: alpha input; P output; beta input
function P = fcn(alpha,beta)

P = diag([5e-2 5e-2 -5e-2]);
